simulink model "gimbal_model_PID_171218v2"  (R2018b)
settings: Solver=VariableStepAuto  StartTime=0.0  StopTime=10  RelTol=1e-3
values from neighbouring files (symbols this model uses):
  DIM = data{4}    [gimbal_dynamics.m]
  DIS = data{5}    [gimbal_dynamics.m]
  F = 5e-5    (= 5e-05)    [BLDC_simulator.m]    (also in engine_parameters.m; engine_parameters_20191210.m = 1)
  I1 = data{1}    [gimbal_dynamics.m]    (also in macierze_inercji.m = sym('I1', [4 4]))
  I2 = data{2}    [gimbal_dynamics.m]    (also in macierze_inercji.m = sym('I2', [4 4]))
  I3 = data{3}    [gimbal_dynamics.m]    (also in macierze_inercji.m = sym('I3', [4 4]))
  J = 7.22e-6    (= 7.22e-06)    [BLDC_simulator.m]    (also in IMU.m = [cos(theta_2)*cos(theta_3) sin(theta_3) 0; engine_parameters.m; engine_parameters_20191210.m = 0.001)
  Kt = 8.44e-3    (= 0.00844)    [BLDC_simulator.m]    (also in engine_parameters.m)
  Kv = 8.44e-3    (= 0.00844)    [BLDC_simulator.m]    (also in engine_parameters.m)
  L = 0.42e-3    (= 0.00042)    [BLDC_simulator.m]    (also in engine_parameters.m; engine_parameters_20191210.m = 0.0005)
  M = [ud_ucz(3:p-1) ud_ucz(3:p-1).^2 ud_ucz(3:p-1).^3 ud_ucz(2:p-2) ud_ucz(2:p-2).^2 ud_ucz(2:p-2).^3 ud_ucz(1:p-3) ud_ucz(1:p-3).^2 ud_ucz(1:p-3).^3 yd_ucz(3:p-1) yd_ucz(3:p-1).^2 yd_ucz(3:p-1).^3 yd_ucz(2:p-2) yd_ucz(2:p-2).^2 yd_ucz(2:p-2).^3 yd_ucz(1:p-3) yd_ucz(1:p-3).^2 yd_ucz(1:p-3).^3]    [Identification_20191023.m]    (also in MI_beta.m = fillmissing(M,'spline'); gimbal_dynamics.m = data{6}; macierze_inercji.m = sym('M', [1 3]))
  R = 7.9    [BLDC_simulator.m]    (also in engine_parameters.m; engine_parameters_20191210.m = 0.5; inversekinematics.m = Rg*Rd*Rm)
libraries: simulink x2
settings Model: Creator=Paweł Tymiński  LastModifiedBy=Paweł Tymiński
settings SFSimCC: SimUseLocalCustomCode=off
settings RTWCC: RTWUseLocalCustomCode=off
settings CodeAppCC: StateflowObjectComments=on
settings SimscapeCC: SimscapeNormalizeSystem=off

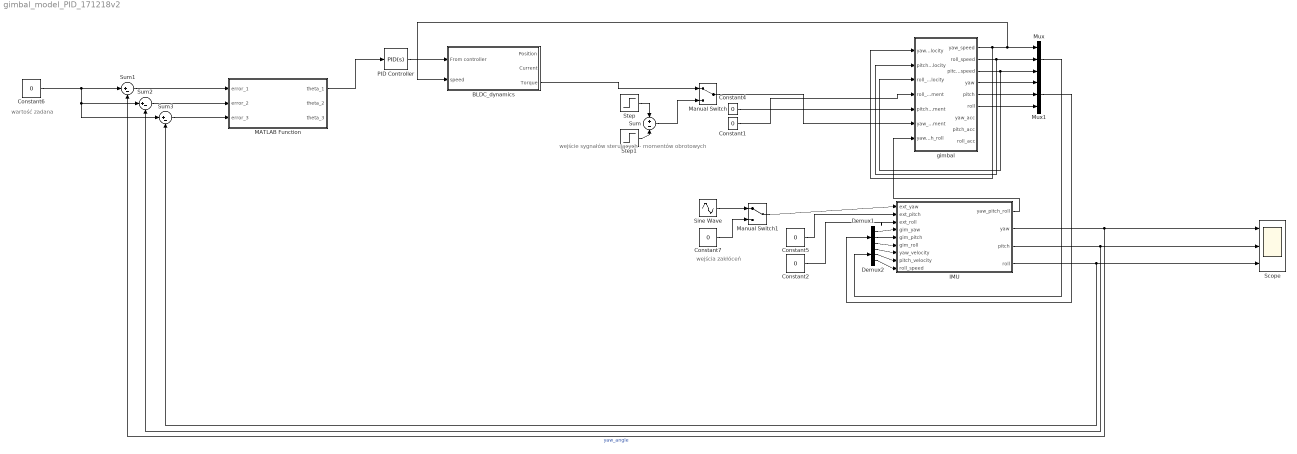
== system gimbal_model_PID_171218v2 ==
  note: wartość zadana
  note: wejście sygnałów sterujących - momentów obrotowych
  note: wejścia zakłóceń
  BLDC_dynamics : Subsystem
  Constant{1..2,4..7} (6 alike) : Constant  Value=0
  Demux1 : Demux  Outputs=3
  Demux2 : Demux  Outputs=3
  IMU : Subsystem
  MATLAB Function : MATLAB Function  TreatAsAtomicUnit=on
  Manual Switch : ManualSwitch
  Manual Switch1 : ManualSwitch
  Mux : Mux  Inputs=3
  Mux1 : Mux  Inputs=3
  PID Controller : simulink/Continuous/PID Controller  Controller=PID  Form=Parallel  TimeDomain=Continuous-time  SampleTime=-1  IntegratorMethod=Forward Euler  FilterMethod=Forward Euler  ControllerParametersSource=internal  P=3.75221520248844  I=9.20583270553454  D=0.233305479962469  UseFilter=on  N=39454.8430256031  TunerSelectOption=Transfer Function Based (PID Tuner App)  InitialConditionSource=internal  InitialConditionForIntegrator=0  InitialConditionForFilter=0  DifferentiatorICPrevScaledInput=0  ExternalReset=none  TrackingMode=off  Kt=1  LimitOutput=off  UpperSaturationLimit=inf  LowerSaturationLimit=-inf  LinearizeAsGain=on  AntiWindupMode=none  Kb=1  POutMin=[]  POutMax=[]  IOutMin=[]  IOutMax=[]  DOutMin=[]  DOutMax=[]  NOutMin=[]  NOutMax=[]  SumOutMin=[]  SumOutMax=[]  SaturationOutMin=[]  SaturationOutMax=[]  PParamMin=[]  PParamMax=[]  IParamMin=[]  IParamMax=[]  DParamMin=[]  DParamMax=[]  NParamMin=[]  NParamMax=[]  KbParamMin=[]  KbParamMax=[]  KtParamMin=[]  KtParamMax=[]  KbOutMin=[]  KbOutMax=[]  KtOutMin=[]  KtOutMax=[]  IntegratorOutMin=[]  IntegratorOutMax=[]  FilterOutMin=[]  FilterOutMax=[]  SumI1OutMin=[]  SumI1OutMax=[]  SumI2OutMin=[]  SumI2OutMax=[]  SumI3OutMin=[]  SumI3OutMax=[]  SumI4OutMin=[]  SumI4OutMax=[]  SumDOutMin=[]  SumDOutMax=[]  DifferentiatorOutMin=[]  DifferentiatorOutMax=[]  FilterDiffOutCoefMin=[]  FilterDiffOutCoefMax=[]  ReciprocalOutMin=[]  ReciprocalOutMax=[]  SumDenOutMin=[]  SumDenOutMax=[]  SumNumOutMin=[]  SumNumOutMax=[]  DivideOutMin=[]  DivideOutMax=[]  IntegratorContinuousStateAttributes=''  IntegratorStateMustResolveToSignalObject=off  IntegratorRTWStateStorageClass=Auto  FilterContinuousStateAttributes=''  FilterStateMustResolveToSignalObject=off  FilterRTWStateStorageClass=Auto  ParallelPVariant=InternalParameters  IdealPVariant=Disabled  IVariant=InternalParameters  DVariant=InternalParameters  IntegratorVariant=Continuous  SatVariant=Disabled  AWVariant=Passthrough  PCopyVariant=Disabled  TRVariant=Disabled  FdbkBlocksVariant=Forward  IdealPFdbkVariant=Disabled  SatFdbkVariant=Disabled  DerivativeFilterVariant=ContFilter  NVariant=InternalParameters  NCopyVariant=Disabled  FilterICVariant=InternalICsFilter  IntegratorICVariant=InternalICs  ExternalResetVariant=Disabled  TRSumVariant=Passthrough  SumFdbkVariant=Disabled  SumVariant=Sum_PID
  Scope : Scope  NumInputPorts=3
  Sine Wave : Sin  SampleTime=0
  Step : Step  SampleTime=0
  Step1 : Step  Time=2  Before=1  After=0  SampleTime=0
  Sum : Sum  Inputs=+-
  Sum1 : Sum  Inputs=|+-
  Sum2 : Sum  Inputs=|+-
  Sum3 : Sum  Inputs=|+-
  gimbal : Subsystem
  wires:
  gimbal/1(yaw_speed) -> gimbal/1(yaw_velocity), BLDC_dynamics/2(speed), Mux/1
  gimbal/3(pitch_speed) -> Mux/3, gimbal/3(roll_velocity)
  gimbal/2(roll_speed) -> Mux/2, gimbal/2(pitch_velocity)
  Mux/1 -> Demux2/1
  Mux1/1 -> Demux1/1
  Demux2/3 -> IMU/9(roll_speed)
  Demux2/2 -> IMU/8(pitch_velocity)
  Demux2/1 -> IMU/7(yaw_velocity)
  Demux1/3 -> IMU/6("gim_roll ")
  Demux1/1 -> IMU/4(gim_yaw)
  Demux1/2 -> IMU/5(gim_pitch)
  IMU/1(yaw_pitch_roll) -> gimbal/7(yaw_pitch_roll)
  Constant2/1 -> IMU/3(ext_roll)
  gimbal/5(pitch) -> Mux1/2
  gimbal/6(roll) -> Mux1/3
  gimbal/4(yaw) -> Mux1/1
  IMU/2(yaw) -> Scope/1, Sum1/2  "yaw_angle"
  IMU/3(pitch) -> Scope/2, Sum2/2
  IMU/4(roll) -> Scope/3, Sum3/2
  Step/1 -> Sum/1
  Step1/1 -> Sum/2
  Constant5/1 -> IMU/2(ext_pitch)
  Sum/1 -> Manual Switch/2
  BLDC_dynamics/3(Torque) -> Manual Switch/1
  Sum3/1 -> MATLAB Function/3(error_3)
  Sum2/1 -> MATLAB Function/2(error_2)
  Sum1/1 -> MATLAB Function/1(error_1)
  Constant6/1 -> Sum3/1, Sum2/1, Sum1/1
  Manual Switch1/1 -> IMU/1(ext_yaw)
  Sine Wave/1 -> Manual Switch1/1
  Constant7/1 -> Manual Switch1/2
  Constant4/1 -> gimbal/5(pitch_moment)
  PID Controller/1 -> BLDC_dynamics/1(From controller)
  MATLAB Function/1(theta_1) -> PID Controller/1
  Manual Switch/1 -> gimbal/6(yaw_moment)
  Constant1/1 -> gimbal/4(roll_moment)

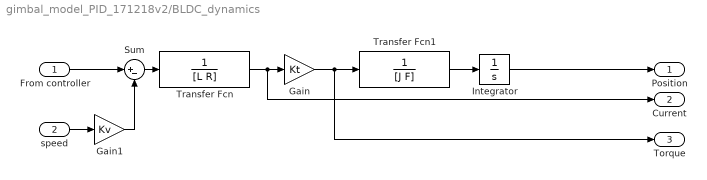
== system gimbal_model_PID_171218v2/BLDC_dynamics ==
  From controller : Inport
  speed : Inport  Port=2
  Gain : Gain  Gain=Kt
  Gain1 : Gain  Gain=Kv
  Integrator : Integrator
  Sum : Sum  Inputs=|+-
  Transfer Fcn : TransferFcn  Denominator=[L R]
  Transfer Fcn1 : TransferFcn  Denominator=[J F]
  Position : Outport
  Current : Outport  Port=2
  Torque : Outport  Port=3
  wires:
  Transfer Fcn1/1 -> Integrator/1
  Transfer Fcn/1 -> Current/1, Gain/1
  Sum/1 -> Transfer Fcn/1
  From controller/1 -> Sum/1
  Gain1/1 -> Sum/2
  Gain/1 -> Transfer Fcn1/1, Torque/1
  Integrator/1 -> Position/1
  speed/1 -> Gain1/1

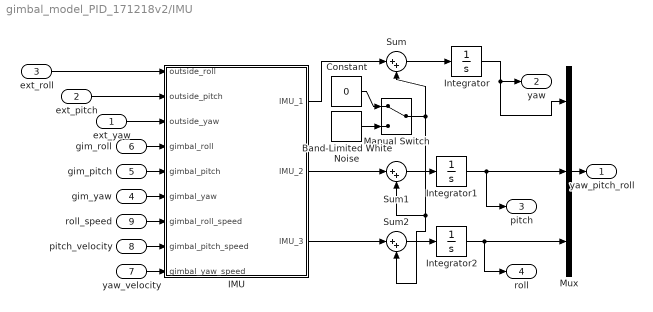
== system gimbal_model_PID_171218v2/IMU ==
  ext_yaw : Inport
  ext_pitch : Inport  Port=2
  ext_roll : Inport  Port=3
  gim_yaw : Inport  Port=4
  gim_pitch : Inport  Port=5
  "gim_roll " : Inport  Port=6
  yaw_velocity : Inport  Port=7
  pitch_velocity : Inport  Port=8
  roll_speed : Inport  Port=9
  Band-Limited White Noise : simulink/Sources/Band-Limited White Noise  Cov=[0.1]  Ts=0.1  seed=[23341]
  Constant : Constant  Value=0
  IMU : MATLAB Function  TreatAsAtomicUnit=on
  Integrator : Integrator
  Integrator1 : Integrator
  Integrator2 : Integrator
  Manual Switch : ManualSwitch
  Mux : Mux  Inputs=3
  Sum : Sum  Inputs=|++
  Sum1 : Sum  Inputs=|++
  Sum2 : Sum  Inputs=|++
  yaw_pitch_roll : Outport
  yaw : Outport  Port=2
  pitch : Outport  Port=3
  roll : Outport  Port=4
  wires:
  roll_speed/1 -> IMU/7(gimbal_roll_speed)
  gim_pitch/1 -> IMU/5(gimbal_pitch)
  Mux/1 -> yaw_pitch_roll/1
  yaw_velocity/1 -> IMU/9(gimbal_yaw_speed)
  IMU/1(IMU_1) -> Sum/1
  pitch_velocity/1 -> IMU/8(gimbal_pitch_speed)
  ext_pitch/1 -> IMU/2(outside_pitch)
  ext_roll/1 -> IMU/1(outside_roll)
  ext_yaw/1 -> IMU/3(outside_yaw)
  "gim_roll "/1 -> IMU/4(gimbal_roll)
  gim_yaw/1 -> IMU/6(gimbal_yaw)
  IMU/3(IMU_3) -> Sum2/1
  IMU/2(IMU_2) -> Sum1/1
  Integrator2/1 -> roll/1, Mux/3
  Manual Switch/1 -> Sum2/2, Sum1/2, Sum/2
  Sum2/1 -> Integrator2/1
  Sum1/1 -> Integrator1/1
  Sum/1 -> Integrator/1
  Integrator1/1 -> pitch/1, Mux/2
  Integrator/1 -> yaw/1, Mux/1
  Band-Limited White Noise/1 -> Manual Switch/2
  Constant/1 -> Manual Switch/1

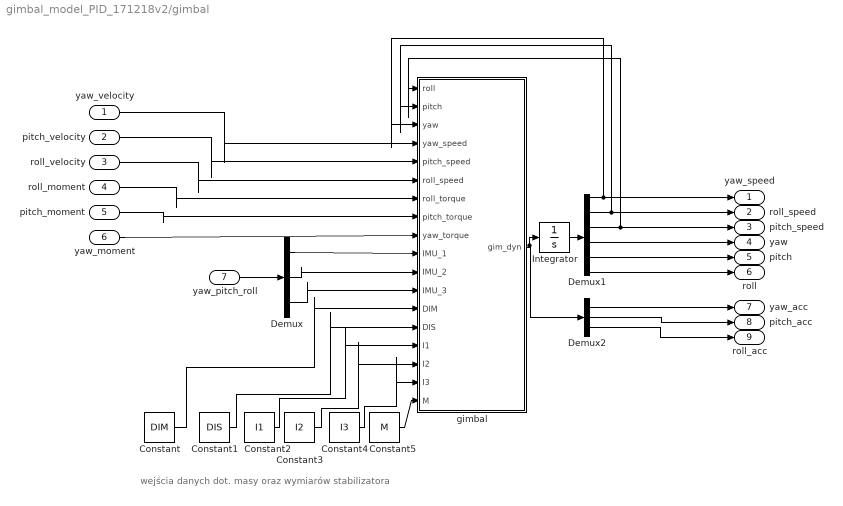
== system gimbal_model_PID_171218v2/gimbal ==
  note: wejścia danych dot. masy oraz wymiarów stabilizatora
  yaw_velocity : Inport
  pitch_velocity : Inport  Port=2
  roll_velocity : Inport  Port=3
  roll_moment : Inport  Port=4
  pitch_moment : Inport  Port=5
  yaw_moment : Inport  Port=6
  yaw_pitch_roll : Inport  Port=7
  Constant : Constant  Value=DIM
  Constant1 : Constant  Value=DIS
  Constant2 : Constant  Value=I1
  Constant3 : Constant  Value=I2
  Constant4 : Constant  Value=I3
  Constant5 : Constant  Value=M
  Demux : Demux  Outputs=3
  Demux1 : Demux  Outputs=6
  Demux2 : Demux  Outputs=3
  Integrator : Integrator
  gimbal : MATLAB Function  TreatAsAtomicUnit=on
  yaw_speed : Outport
  roll_speed : Outport  Port=2
  pitch_speed : Outport  Port=3
  yaw : Outport  Port=4
  pitch : Outport  Port=5
  roll : Outport  Port=6
  yaw_acc : Outport  Port=7
  pitch_acc : Outport  Port=8
  roll_acc : Outport  Port=9
  wires:
  Demux/1 -> gimbal/10(IMU_1)
  Demux/3 -> gimbal/12(IMU_3)
  Demux/2 -> gimbal/11(IMU_2)
  gimbal/1(gim_dyn) -> Demux2/1, Integrator/1
  Demux1/2 -> roll_speed/1, gimbal/2(pitch)
  Demux1/1 -> yaw_speed/1, gimbal/3(yaw)
  yaw_pitch_roll/1 -> Demux/1
  pitch_velocity/1 -> gimbal/5(pitch_speed)
  roll_velocity/1 -> gimbal/6(roll_speed)
  roll_moment/1 -> gimbal/7(roll_torque)
  yaw_velocity/1 -> gimbal/4(yaw_speed)
  yaw_moment/1 -> gimbal/9(yaw_torque)
  pitch_moment/1 -> gimbal/8(pitch_torque)
  Demux1/3 -> pitch_speed/1, gimbal/1(roll)
  Integrator/1 -> Demux1/1
  Demux1/6 -> roll/1
  Demux1/5 -> pitch/1
  Demux1/4 -> yaw/1
  Constant5/1 -> gimbal/18(M)
  Constant4/1 -> gimbal/17(I3)
  Constant3/1 -> gimbal/16(I2)
  Constant2/1 -> gimbal/15(I1)
  Constant1/1 -> gimbal/14(DIS)
  Constant/1 -> gimbal/13(DIM)
  Demux2/1 -> yaw_acc/1
  Demux2/2 -> pitch_acc/1
  Demux2/3 -> roll_acc/1

== matlab function gimbal_model_PID_171218v2/IMU/IMU ==
  data: outside_roll input; IMU_1 output; outside_pitch input; outside_yaw input; gimbal_roll input; gimbal_pitch input; gimbal_yaw input; gimbal_roll_speed input; gimbal_pitch_speed input; gimbal_yaw_speed input; IMU_2 output; IMU_3 output

function [IMU_1, IMU_2, IMU_3] = IMU(outside_roll,outside_pitch,outside_yaw,gimbal_roll , gimbal_pitch , gimbal_yaw , gimbal_roll_speed ,gimbal_pitch_speed , gimbal_yaw_speed )
% kąty gimbala
theta_1 = gimbal_yaw ;
theta_2 = gimbal_pitch ;
theta_3 = gimbal_roll ;

J_0 =[1 0 0;
    0 cos(theta_1) -sin(theta_1);
   -sin(theta_2) cos(theta_2)*sin(theta_1) cos(theta_1)*cos(theta_2)];
Phi_0 = [outside_yaw; outside_pitch; outside_roll];

Omega_phi = J_0*Phi_0;

Omega = [gimbal_yaw_speed; gimbal_pitch_speed; gimbal_roll_speed];

J = [cos(theta_2)*cos(theta_3) sin(theta_3) 0;
    cos(theta_2)*sin(theta_3) cos(theta_3) 0;
    -sin(theta_2) 0 1];
A=J*(Omega_phi + Omega);

IMU_1 = A(1); %yaw
IMU_2 = A(2); %pitch
IMU_3 = A(3); %roll

end

== matlab function gimbal_model_PID_171218v2/MATLAB Function ==
  data: error_1 input; theta_1 output; error_2 input; error_3 input; theta_2 output; theta_3 output
%funkcja kalkulująca nowe nastawy silników na podstawie błędów między
%wartości aktualnych i zadanych 
%Rozdział 2.2.2 "Inverse Kinematics" -
%Modelling and control of an advanced camera gimbal "Jakob Johansson"

function [theta_1,theta_2,theta_3] = fcn(error_1,error_2,error_3)
E=[cos(error_1)*cos(error_3)-sin(error_1)*sin(error_2)*sin(error_3) -cos(error_2)*sin(error_1) cos(error_1)*sin(error_1)+cos(error_3)*sin(error_1)*sin(error_2);
cos(error_3)*sin(error_1)+cos(error_1)*sin(error_2)*sin(error_2) cos(error_1)*cos(error_2) sin(error_1)*sin(error_3)-cos(error_1)*cos(error_3)*sin(error_2);
-cos(error_2)*sin(error_3) sin(error_2) cos(error_2)*cos(error_3)];
r12 = E(1,2);
r22 = E(2,2);
r31 = E(3,1);
r32 = E(3,2);
r33 = E(3,3);
theta_1=atan2(-r12,r22);
theta_2=asin(r32);
theta_3=atan2(-r31,r33);
end

== matlab function gimbal_model_PID_171218v2/gimbal/gimbal ==
  data: roll input; gim_dyn output; pitch input; yaw input; yaw_speed input; pitch_speed input; roll_speed input; roll_torque input; pitch_torque input; yaw_torque input; IMU_1 input; IMU_2 input; IMU_3 input; DIM input; DIS input; I1 input; I2 input; I3 input; M input
%Opis dynamiki stabilizatora w oparciu o wzory wyprowadzone z pracy
%"Stephan von Nispen - Design and control of a three-axis gimbal"



function gim_dyn = gimbal_dynamics(roll,pitch,yaw,yaw_speed,pitch_speed,roll_speed,roll_torque,pitch_torque,yaw_torque,IMU_1,IMU_2,IMU_3,DIM,DIS,I1,I2,I3,M)

%stała grawitacji
g = 9.81;


%-------------ZMIENNE--------------
% odczyty z IMU
alpha_1 = IMU_1;
alpha_2 = IMU_2;
alpha_3 = IMU_3;
IMU = [alpha_1; alpha_2; alpha_3];

% momenty generowane przez silnik - zmienne sterujace
 T1 = yaw_torque ;
 T2 = pitch_torque ;
 T3 = roll_torque ;
%predkosci katowe osiagane przez gimbal
 om_1 = yaw_speed ;
 om_2 = pitch_speed ;
 om_3 = roll_speed ;
Omega = [om_1; om_2; om_3];
%kąty osiagane aktualnie przez gimbal
 theta_1 = yaw ;
 theta_2 = pitch ;
 theta_3 = roll ;
    THETA = [theta_1; theta_2; theta_3];

%---------------FUNKCJE---------------------

H = calculate_H_matrix(THETA,Omega,I1,I2,I3,DIM);
D = calculate_D_matrix(THETA,I1,I2,I3,DIM);
Q = calculate_Q_matrix(T1,T2,T3,Omega);
G = calculate_G_matrix(IMU,THETA,DIM,g,M,DIS);

gim_dyn = [inv(D)\(Q-H-G); Omega];
end
